simulink model "ccam"  (Simulink 7.3)
settings: Solver=ode45  StartTime=0.0  StopTime=2  RelTol=1e-3
libraries: simulink x2
settings Model: Creator=Sainquake  LastModifiedBy=Sainquake Notebook

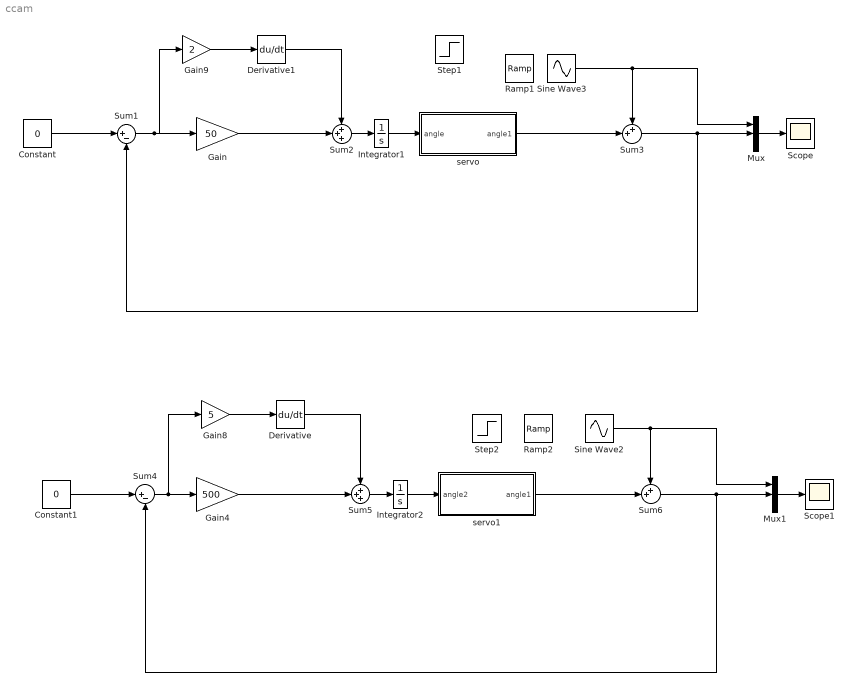
== system ccam ==
  Constant : Constant  Value=0  OutDataType=fixdt(1, 16)  OutScaling=2^0
  Constant1 : Constant  Value=0  OutDataType=fixdt(1, 16)  OutScaling=2^0
  Derivative : Derivative
  Derivative1 : Derivative
  Gain : Gain  Gain=50  ParameterDataType=fixdt(1, 16)  ParameterScaling=2^0  OutDataType=fixdt(1, 16)  OutScaling=2^0
  Gain4 : Gain  Gain=500  ParameterDataType=fixdt(1, 16)  ParameterScaling=2^0  OutDataType=fixdt(1, 16)  OutScaling=2^0
  Gain8 : Gain  Gain=5  ParameterDataType=fixdt(1, 16)  ParameterScaling=2^0  OutDataType=fixdt(1, 16)  OutScaling=2^0
  Gain9 : Gain  Gain=2  ParameterDataType=fixdt(1, 16)  ParameterScaling=2^0  OutDataType=fixdt(1, 16)  OutScaling=2^0
  Integrator1 : Integrator
  Integrator2 : Integrator
  Mux : Mux  Inputs=3
  Mux1 : Mux  Inputs=3
  Ramp1 : simulink/Sources/Ramp  SystemSampleTime=-1  slope=100  start=1  X0=0
  Ramp2 : simulink/Sources/Ramp  SystemSampleTime=-1  slope=100  start=1  X0=0
  Scope : Scope
  Scope1 : Scope
      settings: SaveName=ScopeData2
  Sine Wave2 : Sin  Amplitude=20  Bias=0  Frequency=sqrt(9.8/2)  Phase=0  Samples=10  SampleTime=0  Offset=0
  Sine Wave3 : Sin  Amplitude=20  Bias=0  Frequency=sqrt(9.8/0.9)  Phase=0  Samples=10  SampleTime=0  Offset=0
  Step1 : Step  After=60  SampleTime=0
  Step2 : Step  After=60  SampleTime=0
  Sum1 : Sum  Inputs=|+-  OutDataType=fixdt(1, 16)  OutScaling=2^0
  Sum2 : Sum  Inputs=+++  OutDataType=fixdt(1, 16)  OutScaling=2^0
  Sum3 : Sum  Inputs=++|  OutDataType=fixdt(1, 16)  OutScaling=2^0
  Sum4 : Sum  Inputs=|+-  OutDataType=fixdt(1, 16)  OutScaling=2^0
  Sum5 : Sum  Inputs=+++  OutDataType=fixdt(1, 16)  OutScaling=2^0
  Sum6 : Sum  Inputs=++|  OutDataType=fixdt(1, 16)  OutScaling=2^0
  servo : Subsystem
  servo1 : Subsystem
  wires:
  Constant/1 -> Sum1/1
  Sum1/1 -> Gain9/1, Gain/1
  Mux/1 -> Scope/1
  Sum3/1 -> Mux/2, Sum1/2
  Sine Wave3/1 -> Sum3/1, Mux/1
  Gain/1 -> Sum2/2
  servo/1(angle1) -> Sum3/2
  Integrator1/1 -> servo/1(angle)
  Constant1/1 -> Sum4/1
  Sum4/1 -> Gain4/1, Gain8/1
  Sum5/1 -> Integrator2/1
  Mux1/1 -> Scope1/1
  Sum6/1 -> Mux1/2, Sum4/2
  Sine Wave2/1 -> Sum6/1, Mux1/1
  Gain4/1 -> Sum5/2
  servo1/1(angle1) -> Sum6/2
  Integrator2/1 -> servo1/1(angle2)
  Derivative/1 -> Sum5/1
  Gain8/1 -> Derivative/1
  Derivative1/1 -> Sum2/1
  Gain9/1 -> Derivative1/1
  Sum2/1 -> Integrator1/1

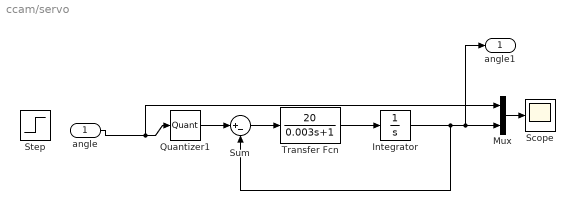
== system ccam/servo ==
  angle : Inport  OutDataType=fixdt(1, 16)  OutScaling=2^0
  Integrator : Integrator
  Mux : Mux  Inputs=3
  Quantizer1 : Quantizer  QuantizationInterval=1  SampleTime=0.02
  Scope : Scope
  Step : Step  Time=0.2  After=60  SampleTime=0
  Sum : Sum  Inputs=|+-  OutDataType=fixdt(1, 16)  OutScaling=2^0
  Transfer Fcn : TransferFcn  Numerator=[20]  Denominator=[0.003 1]
  angle1 : Outport  OutDataType=fixdt(1, 16)  OutScaling=2^0
  wires:
  Sum/1 -> Transfer Fcn/1
  Quantizer1/1 -> Sum/1
  Integrator/1 -> Sum/2, Mux/3, angle1/1
  Mux/1 -> Scope/1
  Transfer Fcn/1 -> Integrator/1
  angle/1 -> Quantizer1/1, Mux/1

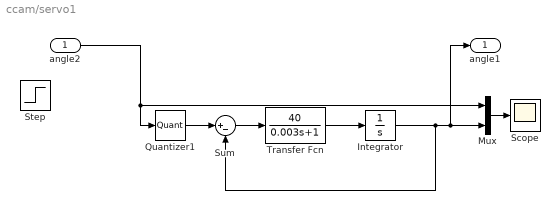
== system ccam/servo1 ==
  angle2 : Inport  OutDataType=fixdt(1, 16)  OutScaling=2^0
  Integrator : Integrator
  Mux : Mux  Inputs=3
  Quantizer1 : Quantizer  QuantizationInterval=1  SampleTime=0.002
  Scope : Scope
  Step : Step  Time=0.1  After=60  SampleTime=0
  Sum : Sum  Inputs=|+-  OutDataType=fixdt(1, 16)  OutScaling=2^0
  Transfer Fcn : TransferFcn  Numerator=[40]  Denominator=[0.003 1]
  angle1 : Outport  OutDataType=fixdt(1, 16)  OutScaling=2^0
  wires:
  Sum/1 -> Transfer Fcn/1
  Quantizer1/1 -> Sum/1
  Integrator/1 -> Sum/2, Mux/3, angle1/1
  Mux/1 -> Scope/1
  angle2/1 -> Quantizer1/1, Mux/1
  Transfer Fcn/1 -> Integrator/1
